simulink model "asger_1_simulink"  (R2017b)
settings: Solver=VariableStepAuto  StartTime=0.0  StopTime=100.0  RelTol=1e-3
values from neighbouring files (symbols this model uses):
  alpha = 0.7    [asger_1.m]
  b = 0.5    [asger_1.m]
  Kp = 1/M    [asger_1.m]
  tau = 10    [asger_1.m]
  tau_d = 1/(wc*sqrt(alpha))    [asger_1.m]
  tau_i = Ni/wc    (= 0.819672131148)    [asger_1.m]
settings Model: Creator=asger  LastModifiedBy=asger

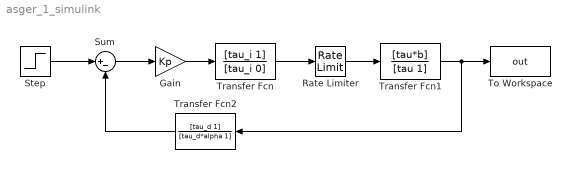
== system asger_1_simulink ==
  Gain : Gain  Gain=Kp
  Rate Limiter : RateLimiter
  Step : Step  Time=0  After=3  SampleTime=0
  Sum : Sum  Inputs=|+-
  To Workspace : ToWorkspace  VariableName=out  SaveFormat=Timeseries  SampleTime=-1
  Transfer Fcn : TransferFcn  Numerator=[tau_i 1]  Denominator=[tau_i 0]
  Transfer Fcn1 : TransferFcn  Numerator=[tau*b]  Denominator=[tau 1]
  Transfer Fcn2 : TransferFcn  Numerator=[tau_d 1]  Denominator=[tau_d*alpha 1]
  wires:
  Sum/1 -> Gain/1
  Step/1 -> Sum/1
  Transfer Fcn1/1 -> Transfer Fcn2/1, To Workspace/1
  Transfer Fcn2/1 -> Sum/2
  Rate Limiter/1 -> Transfer Fcn1/1
  Transfer Fcn/1 -> Rate Limiter/1
  Gain/1 -> Transfer Fcn/1
